simulink model "BaseModel"  (R2020b)
settings: Solver=VariableStepAuto  StartTime=0.0  StopTime=10.0  RelTol=1e-3
settings Model: Creator=huessyjo  LastModifiedBy=huessyjo

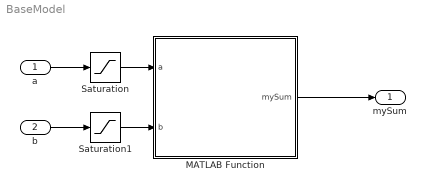
== system BaseModel ==
  a : Inport
  b : Inport  Port=2
  MATLAB Function : MATLAB Function  TreatAsAtomicUnit=on
  Saturation : Saturate  UpperLimit=1  LowerLimit=0
  Saturation1 : Saturate  UpperLimit=1  LowerLimit=0
  mySum : Outport
  wires:
  a/1 -> Saturation/1
  b/1 -> Saturation1/1
  Saturation/1 -> MATLAB Function/1(a)
  Saturation1/1 -> MATLAB Function/2(b)
  MATLAB Function/1(mySum) -> mySum/1

== matlab function BaseModel/MATLAB Function ==
  data: a input; mySum output; b input
function mySum  = myCalculator(a,b)

mySum  = a+b;
